simulink model "fmu_simulation"  (R2024a)
settings: Solver=ode1  StartTime=0.0  StopTime=200.0  FixedStep=0.01  RelTol=1e-3
settings Model: Creator=rkhan  LastModifiedBy=rkhan

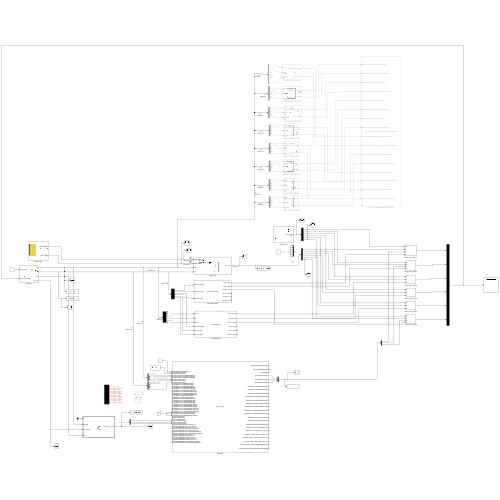
[thumbnail: Simulink's stored preview of the top-level diagram]
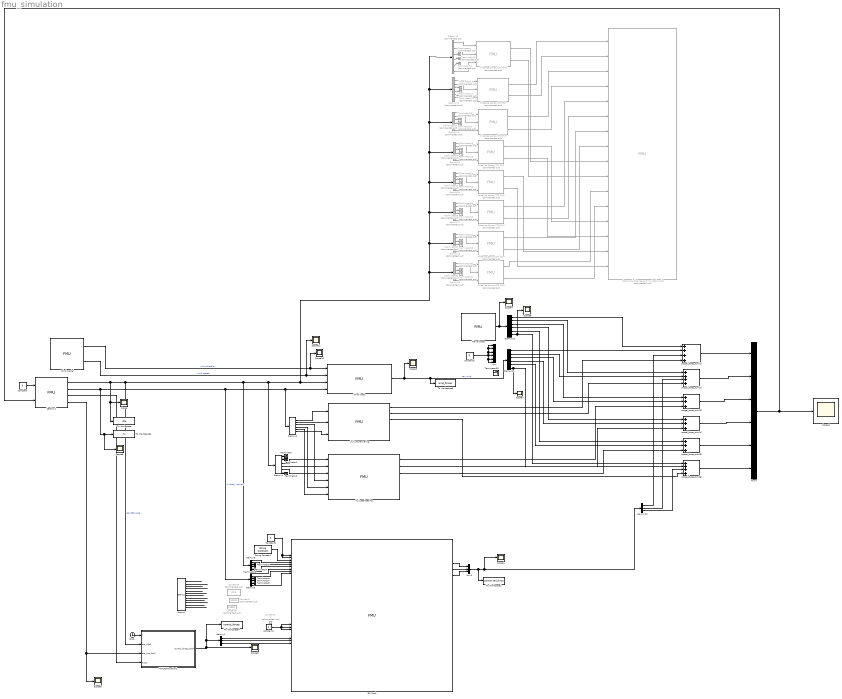
== system fmu_simulation ==
  Clock : Clock
  Constant : Constant  Value=0  OutDataTypeStr=boolean
  Constant1 : Constant  Value=0
  Constant2 : Constant  OutDataTypeStr=boolean
  Constant3 : Constant  Commented=on  Value=0
  Constant4 : Constant  OutDataTypeStr=double
  Constant6 : Constant  Commented=on  Value=3.0508
  Constant7 : Constant  Commented=on  Value=494.9
  Constant8 : Constant  Commented=on  Value=87.5
  DP Mock : FMU  FMUName=fmi_dp_mock.fmu  FMUMode=CoSimulation  FMUInitializeEnumObject=off  FMUCachedDialogLayout="{\"Geometry\":[471,-1082,1182,943],\"ParameterColumnsWidthConfig\":\"{\\\"columns\\\":[{\\\"name\\\":\\\"Parameter\\\",\\\"width\\\":422},{\\\"name\\\":\\\"Value\\\",\\\"width\\\":287},{\\\"name\\\":\\\"Unit\\\",\\\"width\\\":277},{\\\"name\\\":\\\"Description\\\",\\\"width\\\":339}]}\",\"InputColumnsWidthConfig\":[],\"OutputColumnsWidthConfig\":[]}"  Kp_0_=1485  Kp_1_=1800  Kp_2_=100000  Ki_0_=74  Ki_1_=90  Ki_2_=657  Kd_0_=19700  Kd_1_=23000  Kd_2_=173000  GeneralizedForcesSaturation_0_=10000  GeneralizedForcesSaturation_1_=10000  GeneralizedForcesSaturation_2_=35000  IntegralActionSaturation_0_=1000  IntegralActionSaturation_1_=1000  IntegralActionSaturation_2_=5000  MassMatrixDiagonal_0_=16500  MassMatrixDiagonal_1_=20000  MassMatrixDiagonal_2_=146000  DampingMatrixDiagonal_0_=100  DampingMatrixDiagonal_1_=1000  DampingMatrixDiagonal_2_=2200  MaxEffort_0_=5000  MaxEffort_1_=5000  MaxEffort_2_=5000  autopilot_heading_pid_Kp=70000  autopilot_heading_pid_Ki=0  autopilot_heading_pid_Kd=100000  autopilot_surge_speed_pid_Kp=3000  autopilot_surge_speed_pid_Ki=50  autopilot_surge_speed_pid_Kd=1000  mask(fmi_dp_mock [Co-Simulation, v2.0]){}
      mask Display:
      | disp('fmi_dp_mock');
      | port_label('output',1,'readyForAutonomyEnabled');
      | port_label('output',2,'autonomyModeEnabled');
      | port_label('output',3,'controlMode');
      | port_label('output',4,'generalizedForces[0]');
      | port_label('output',5,'generalizedForces[1]');
      | port_label('output',6,'generalizedForces[2]');
      | port_label('output',7,'refDPActive.northEastHeading[0]');
      | port_label('output',8,'refDPActive.northEastHeading[1]');
      | port_label('output',9,'refDPActive.northEastHeading[2]');
      | port_label('output',10,'refDPActive.northEastHeadingVel[0]');
      | port_label('output',11,'refDPActive.northEastHeadingVel[1]');
      | port_label('output',12,'refDPActive.northEastHeadingVel[2]');
      | port_label('output',13,'refDPActive.northEastHeadingAccel[0]');
      | port_label('output',14,'refDPActive.northEastHeadingAccel[1]');
      | port_label('output',15,'refDPActive.northEastHeadingAccel[2]');
      | port_label('output',16,'refDPActive.surgeIntegratorMode');
      | port_label('output',17,'refDPActive.swayIntegratorMode');
      | port_label('output',18,'refDPActive.headingIntegratorMode');
      | port_label('output',19,'autopilot_active_inputs.heading_ref');
      | port_label('output',20,'autopilot_active_inputs.yaw_rate_ref');
      | port_label('output',21,'autopilot_active_inputs.yaw_accel_ref');
      | port_label('output',22,'autopilot_active_inputs.surge_speed_ref');
      | port_label('output',23,'autopilot_active_inputs.surge_accel_ref');
      | port_label('output',24,'autopilot_active_inputs.surgeIntegratorMode');
      | port_label('output',25,'autopilot_active_inputs.headingIntegratorMode');
      | port_label('input',1,'enableReadyForAutonomy');
      | port_label('input',2,'enableAutonomyMode');
      | port_label('input',3,'desiredControlMode');
      | port_label('input',4,'measurements.northEastHeading[0]');
      | port_label('input',5,'measurements.northEastHeading[1]');
      | port_label('input',6,'measurements.northEastHeading[2]');
      | port_label('input',7,'measurements.nu[0]');
      | port_label('input',8,'measurements.nu[1]');
      | port_label('input',9,'measurements.nu[2]');
      | port_label('input',10,'refDpManual.northEastHeading[0]');
      | port_label('input',11,'refDpManual.northEastHeading[1]');
      | port_label('input',12,'refDpManual.northEastHeading[2]');
      | port_label('input',13,'refDpManual.northEastHeadingVel[0]');
      | port_label('input',14,'refDpManual.northEastHeadingVel[1]');
      | port_label('input',15,'refDpManual.northEastHeadingVel[2]');
      | port_label('input',16,'refDpManual.northEastHeadingAccel[0]');
      | port_label('input',17,'refDpManual.northEastHeadingAccel[1]');
      | port_label('input',18,'refDpManual.northEastHeadingAccel[2]');
      | port_label('input',19,'refDpManual.surgeIntegratorMode');
      | port_label('input',20,'refDpManual.swayIntegratorMode');
      | port_label('input',21,'refDpManual.headingIntegratorMode');
      | port_label('input',22,'refDpAutonomy.northEastHeading[0]');
      | port_label('input',23,'refDpAutonomy.northEastHeading[1]');
      | port_label('input',24,'refDpAutonomy.northEastHeading[2]');
      | port_label('input',25,'refDpAutonomy.northEastHeadingVel[0]');
      | port_label('input',26,'refDpAutonomy.northEastHeadingVel[1]');
      | port_label('input',27,'refDpAutonomy.northEastHeadingVel[2]');
      | port_label('input',28,'refDpAutonomy.northEastHeadingAccel[0]');
      | port_label('input',29,'refDpAutonomy.northEastHeadingAccel[1]');
      | port_label('input',30,'refDpAutonomy.northEastHeadingAccel[2]');
      | port_label('input',31,'refDpAutonomy.surgeIntegratorMode');
      | port_label('input',32,'refDpAutonomy.swayIntegratorMode');
      | port_label('input',33,'refDpAutonomy.headingIntegratorMode');
      | port_label('input',34,'refForcesManual[0]');
      | port_label('input',35,'refForcesManual[1]');
      | port_label('input',36,'refForcesManual[2]');
      | port_label('input',37,'refForcesAutonomy[0]');
      | port_label('input',38,'refForcesAutonomy[1]');
      | port_label('input',39,'refForcesAutonomy[2]');
      | port_label('input',40,'autopilotInputsAutonomy.heading_ref');
      | port_label('input',41,'autopilotInputsAutonomy.yaw_rate_ref');
      | port_label('input',42,'autopilotInputsAutonomy.yaw_accel_ref');
      | port_label('input',43,'autopilotInputsAutonomy.surge_speed_ref');
      | port_label('input',44,'autopilotInputsAutonomy.surge_accel_ref');
      | port_label('input',45,'autopilotInputsAutonomy.surgeIntegratorMode');
      | port_label('input',46,'autopilotInputsAutonomy.headingIntegratorMode');
      | port_label('input',47,'autopilotInputsManual.heading_ref');
      | port_label('input',48,'autopilotInputsManual.yaw_rate_ref');
      | port_label('input',49,'autopilotInputsManual.yaw_accel_ref');
      | port_label('input',50,'autopilotInputsManual.surge_speed_ref');
      | port_label('input',51,'autopilotInputsManual.surge_accel_ref');
      | port_label('input',52,'autopilotInputsManual.surgeIntegratorMode');
      | port_label('input',53,'autopilotInputsManual.headingIntegratorMode');
  Demux : Demux  Outputs=12
  Demux1 : Demux  Outputs=3
  Demux{12..19} (8 alike) : Demux  Commented=on  Outputs=6
  Demux{3..6,20..21} (6 alike) : Demux  Outputs=6
  Demux22 : Demux  Outputs=3
  Distance Sensor ZT1 FS-S : FMU  Commented=on  FMUName=UltrasonicDistanceSensor.fmu  FMUMode=CoSimulation  FMUCreateBusObject=off  FMUInitializeEnumObject=off  max_range=2  min_range=0.15  quay_1_depth=4.8  quay_1_p0=[81.7373060391681 498.883639455798]  quay_1_p1=[80.9216766435735 489.920674059846]  quay_2_depth=0.71  quay_2_p0=[93.6113480294073 496.95461073283]  quay_2_p1=[81.6607275014706 498.042116593623]  quay_3_depth=4.8  quay_3_p0=[619.016624410391 129.501263835181]  quay_3_p1=[618.965112725514 141.501153274102]  quay_4_depth=0.71  quay_4_p0=[606.991215224254 135.394697376503]  quay_4_p1=[618.991104663175 135.44620906138]  sensor_pose_psi=1.5708  sensor_pose_x=4.913  sensor_pose_y=2.4487  quay_1_en=on  quay_2_en=on  quay_3_en=on  quay_4_en=on  mask(UltrasonicDistanceSensor [Co-Simulation, v2.0]){}
      mask Display:
      | if (exist([Simulink.fileGenControl('get','CacheFolder') '\slprj\_fmu\777984f43c50f29a2c3e45720daf4c20\UltrasonicDistanceSensor\model.png'],'file'))
      |     image([Simulink.fileGenControl('get','CacheFolder') '\slprj\_fmu\777984f43c50f29a2c3e45720daf4c20\UltrasonicDistanceSensor\model.png']);
      | else
      |     disp('UltrasonicDistanceSensor');
      | end
      | port_label('output',1,'distance_measurement');
      | port_label('output',2,'signal_valid');
      | port_label('input',1,'north');
      | port_label('input',2,'east');
      | port_label('input',3,'heading');
  Distance Sensor ZT2 FS-F : FMU  Commented=on  FMUName=UltrasonicDistanceSensor_1.fmu  FMUMode=CoSimulation  FMUCreateBusObject=off  FMUInitializeEnumObject=off  max_range=2  min_range=0.15  quay_1_depth=4.8  quay_1_p0=[81.7373060391681 498.883639455798]  quay_1_p1=[80.9216766435735 489.920674059846]  quay_2_depth=0.71  quay_2_p0=[93.6113480294073 496.95461073283]  quay_2_p1=[81.6607275014706 498.042116593623]  quay_3_depth=4.8  quay_3_p0=[619.016624410391 129.501263835181]  quay_3_p1=[618.965112725514 141.501153274102]  quay_4_depth=0.71  quay_4_p0=[606.991215224254 135.394697376503]  quay_4_p1=[618.991104663175 135.44620906138]  sensor_pose_psi=0  sensor_pose_x=5.9479  sensor_pose_y=1.5  quay_1_en=on  quay_2_en=on  quay_3_en=on  quay_4_en=on  mask(UltrasonicDistanceSensor_1 [Co-Simulation, v2.0]){}
      mask Display:
      | if (exist([Simulink.fileGenControl('get','CacheFolder') '\slprj\_fmu\d35cb4a80b2d73ab213e5ce7f852a3cb\UltrasonicDistanceSensor_1\model.png'],'file'))
      |     image([Simulink.fileGenControl('get','CacheFolder') '\slprj\_fmu\d35cb4a80b2d73ab213e5ce7f852a3cb\UltrasonicDistanceSensor_1\model.png']);
      | else
      |     disp('UltrasonicDistanceSensor_1');
      | end
      | port_label('output',1,'distance_measurement');
      | port_label('output',2,'signal_valid');
      | port_label('input',1,'north');
      | port_label('input',2,'east');
      | port_label('input',3,'heading');
  Distance Sensor ZT3 FP-F : FMU  Commented=on  FMUName=UltrasonicDistanceSensor_2.fmu  FMUMode=CoSimulation  FMUCreateBusObject=off  FMUInitializeEnumObject=off  max_range=2  min_range=0.15  quay_1_depth=4.8  quay_1_p0=[81.7373060391681 498.883639455798]  quay_1_p1=[80.9216766435735 489.920674059846]  quay_2_depth=0.71  quay_2_p0=[93.6113480294073 496.95461073283]  quay_2_p1=[81.6607275014706 498.042116593623]  quay_3_depth=4.8  quay_3_p0=[619.016624410391 129.501263835181]  quay_3_p1=[618.965112725514 141.501153274102]  quay_4_depth=0.71  quay_4_p0=[606.991215224254 135.394697376503]  quay_4_p1=[618.991104663175 135.44620906138]  sensor_pose_psi=0  sensor_pose_x=5.9465  sensor_pose_y=-1.5  quay_1_en=on  quay_2_en=on  quay_3_en=on  quay_4_en=on  mask(UltrasonicDistanceSensor_2 [Co-Simulation, v2.0]){}
      mask Display:
      | if (exist([Simulink.fileGenControl('get','CacheFolder') '\slprj\_fmu\12532f91765f62f696db53de24741f0c\UltrasonicDistanceSensor_2\model.png'],'file'))
      |     image([Simulink.fileGenControl('get','CacheFolder') '\slprj\_fmu\12532f91765f62f696db53de24741f0c\UltrasonicDistanceSensor_2\model.png']);
      | else
      |     disp('UltrasonicDistanceSensor_2');
      | end
      | port_label('output',1,'distance_measurement');
      | port_label('output',2,'signal_valid');
      | port_label('input',1,'north');
      | port_label('input',2,'east');
      | port_label('input',3,'heading');
  Distance Sensor ZT4 FP-P : FMU  Commented=on  FMUName=UltrasonicDistanceSensor_3.fmu  FMUMode=CoSimulation  FMUCreateBusObject=off  FMUInitializeEnumObject=off  max_range=2  min_range=0.15  quay_1_depth=4.8  quay_1_p0=[81.7373060391681 498.883639455798]  quay_1_p1=[80.9216766435735 489.920674059846]  quay_2_depth=0.71  quay_2_p0=[93.6113480294073 496.95461073283]  quay_2_p1=[81.6607275014706 498.042116593623]  quay_3_depth=4.8  quay_3_p0=[619.016624410391 129.501263835181]  quay_3_p1=[618.965112725514 141.501153274102]  quay_4_depth=0.71  quay_4_p0=[606.991215224254 135.394697376503]  quay_4_p1=[618.991104663175 135.44620906138]  sensor_pose_psi=-1.5708  sensor_pose_x=4.913  sensor_pose_y=-2.4527  quay_1_en=on  quay_2_en=on  quay_3_en=on  quay_4_en=on  mask(UltrasonicDistanceSensor_3 [Co-Simulation, v2.0]){}
      mask Display:
      | if (exist([Simulink.fileGenControl('get','CacheFolder') '\slprj\_fmu\33e4b1bd19c1a4bbf282549265bfa70a\UltrasonicDistanceSensor_3\model.png'],'file'))
      |     image([Simulink.fileGenControl('get','CacheFolder') '\slprj\_fmu\33e4b1bd19c1a4bbf282549265bfa70a\UltrasonicDistanceSensor_3\model.png']);
      | else
      |     disp('UltrasonicDistanceSensor_3');
      | end
      | port_label('output',1,'distance_measurement');
      | port_label('output',2,'signal_valid');
      | port_label('input',1,'north');
      | port_label('input',2,'east');
      | port_label('input',3,'heading');
  Distance Sensor ZT5 AP-P : FMU  Commented=on  FMUName=UltrasonicDistanceSensor_4.fmu  FMUMode=CoSimulation  FMUCreateBusObject=off  FMUInitializeEnumObject=off  max_range=2  min_range=0.15  quay_1_depth=4.8  quay_1_p0=[81.7373060391681 498.883639455798]  quay_1_p1=[80.9216766435735 489.920674059846]  quay_2_depth=0.71  quay_2_p0=[93.6113480294073 496.95461073283]  quay_2_p1=[81.6607275014706 498.042116593623]  quay_3_depth=4.8  quay_3_p0=[619.016624410391 129.501263835181]  quay_3_p1=[618.965112725514 141.501153274102]  quay_4_depth=0.71  quay_4_p0=[606.991215224254 135.394697376503]  quay_4_p1=[618.991104663175 135.44620906138]  sensor_pose_psi=-1.5708  sensor_pose_x=-4.913  sensor_pose_y=-2.4514  quay_1_en=on  quay_2_en=on  quay_3_en=on  quay_4_en=on  mask(UltrasonicDistanceSensor_4 [Co-Simulation, v2.0]){}
      mask Display:
      | if (exist([Simulink.fileGenControl('get','CacheFolder') '\slprj\_fmu\2c6022cae16bfe16619e246ed39a73a9\UltrasonicDistanceSensor_4\model.png'],'file'))
      |     image([Simulink.fileGenControl('get','CacheFolder') '\slprj\_fmu\2c6022cae16bfe16619e246ed39a73a9\UltrasonicDistanceSensor_4\model.png']);
      | else
      |     disp('UltrasonicDistanceSensor_4');
      | end
      | port_label('output',1,'distance_measurement');
      | port_label('output',2,'signal_valid');
      | port_label('input',1,'north');
      | port_label('input',2,'east');
      | port_label('input',3,'heading');
  Distance Sensor ZT6 AP-A : FMU  Commented=on  FMUName=UltrasonicDistanceSensor_5.fmu  FMUMode=CoSimulation  FMUCreateBusObject=off  FMUInitializeEnumObject=off  max_range=2  min_range=0.15  quay_1_depth=4.8  quay_1_p0=[81.7373060391681 498.883639455798]  quay_1_p1=[80.9216766435735 489.920674059846]  quay_2_depth=0.71  quay_2_p0=[93.6113480294073 496.95461073283]  quay_2_p1=[81.6607275014706 498.042116593623]  quay_3_depth=4.8  quay_3_p0=[619.016624410391 129.501263835181]  quay_3_p1=[618.965112725514 141.501153274102]  quay_4_depth=0.71  quay_4_p0=[606.991215224254 135.394697376503]  quay_4_p1=[618.991104663175 135.44620906138]  sensor_pose_psi=3.1416  sensor_pose_x=-5.9427  sensor_pose_y=-1.5  quay_1_en=on  quay_2_en=on  quay_3_en=on  quay_4_en=on  mask(UltrasonicDistanceSensor_5 [Co-Simulation, v2.0]){}
      mask Display:
      | if (exist([Simulink.fileGenControl('get','CacheFolder') '\slprj\_fmu\5972c6e08933a554bbec62f557174caa\UltrasonicDistanceSensor_5\model.png'],'file'))
      |     image([Simulink.fileGenControl('get','CacheFolder') '\slprj\_fmu\5972c6e08933a554bbec62f557174caa\UltrasonicDistanceSensor_5\model.png']);
      | else
      |     disp('UltrasonicDistanceSensor_5');
      | end
      | port_label('output',1,'distance_measurement');
      | port_label('output',2,'signal_valid');
      | port_label('input',1,'north');
      | port_label('input',2,'east');
      | port_label('input',3,'heading');
  Distance Sensor ZT7 AS-A : FMU  Commented=on  FMUName=UltrasonicDistanceSensor_6.fmu  FMUMode=CoSimulation  FMUCreateBusObject=off  FMUInitializeEnumObject=off  max_range=2  min_range=0.15  quay_1_depth=4.8  quay_1_p0=[81.7373060391681 498.883639455798]  quay_1_p1=[80.9216766435735 489.920674059846]  quay_2_depth=0.71  quay_2_p0=[93.6113480294073 496.95461073283]  quay_2_p1=[81.6607275014706 498.042116593623]  quay_3_depth=4.8  quay_3_p0=[619.016624410391 129.501263835181]  quay_3_p1=[618.965112725514 141.501153274102]  quay_4_depth=0.71  quay_4_p0=[606.991215224254 135.394697376503]  quay_4_p1=[618.991104663175 135.44620906138]  sensor_pose_psi=3.1416  sensor_pose_x=-5.946  sensor_pose_y=1.5  quay_1_en=on  quay_2_en=on  quay_3_en=on  quay_4_en=on  mask(UltrasonicDistanceSensor_6 [Co-Simulation, v2.0]){}
      mask Display:
      | if (exist([Simulink.fileGenControl('get','CacheFolder') '\slprj\_fmu\76e2b9015701c0cf85d1e0a29a928fe7\UltrasonicDistanceSensor_6\model.png'],'file'))
      |     image([Simulink.fileGenControl('get','CacheFolder') '\slprj\_fmu\76e2b9015701c0cf85d1e0a29a928fe7\UltrasonicDistanceSensor_6\model.png']);
      | else
      |     disp('UltrasonicDistanceSensor_6');
      | end
      | port_label('output',1,'distance_measurement');
      | port_label('output',2,'signal_valid');
      | port_label('input',1,'north');
      | port_label('input',2,'east');
      | port_label('input',3,'heading');
  Distance Sensor ZT8 AS-S : FMU  Commented=on  FMUName=UltrasonicDistanceSensor_7.fmu  FMUMode=CoSimulation  FMUCreateBusObject=off  FMUInitializeEnumObject=off  max_range=2  min_range=0.15  quay_1_depth=4.8  quay_1_p0=[81.7373060391681 498.883639455798]  quay_1_p1=[80.9216766435735 489.920674059846]  quay_2_depth=0.71  quay_2_p0=[93.6113480294073 496.95461073283]  quay_2_p1=[81.6607275014706 498.042116593623]  quay_3_depth=4.8  quay_3_p0=[619.016624410391 129.501263835181]  quay_3_p1=[618.965112725514 141.501153274102]  quay_4_depth=0.71  quay_4_p0=[606.991215224254 135.394697376503]  quay_4_p1=[618.991104663175 135.44620906138]  sensor_pose_psi=1.5708  sensor_pose_x=-4.913  sensor_pose_y=2.4532  quay_1_en=on  quay_2_en=on  quay_3_en=on  quay_4_en=on  mask(UltrasonicDistanceSensor_7 [Co-Simulation, v2.0]){}
      mask Display:
      | if (exist([Simulink.fileGenControl('get','CacheFolder') '\slprj\_fmu\fcc687ec8d3596fcafe8ed7ad9aa01b3\UltrasonicDistanceSensor_7\model.png'],'file'))
      |     image([Simulink.fileGenControl('get','CacheFolder') '\slprj\_fmu\fcc687ec8d3596fcafe8ed7ad9aa01b3\UltrasonicDistanceSensor_7\model.png']);
      | else
      |     disp('UltrasonicDistanceSensor_7');
      | end
      | port_label('output',1,'distance_measurement');
      | port_label('output',2,'signal_valid');
      | port_label('input',1,'north');
      | port_label('input',2,'east');
      | port_label('input',3,'heading');
  MATLAB Function1 : MATLAB Function  TreatAsAtomicUnit=on
  Mux : Mux  Inputs=6
  Mux3 : Mux  Inputs=3
  Mux4 : Mux  Inputs=6
  Scope{,1..11} (12 alike) : Scope
  String Constant : StringConstant  String="\"JOYSTICK\""
  Terminator{,1..8,33} (10 alike) : Terminator
  Terminator{9..32} (24 alike) : Terminator  Commented=on
  To Workspace : ToWorkspace  VariableName=eta  SaveFormat=Timeseries  SampleTime=-1
  To Workspace1 : ToWorkspace  VariableName=generalized_forces  SaveFormat=Timeseries  SampleTime=-1
  To Workspace2 : ToWorkspace  VariableName=nu  SaveFormat=Timeseries  SampleTime=-1
  To Workspace3 : ToWorkspace  VariableName=wind_forces  SaveFormat=Structure With Time  SampleTime=-1
  To Workspace4 : ToWorkspace  VariableName=control_forces  SaveFormat=Timeseries  SampleTime=-1
  Wave forces : FMU  FMUName=wave_forces.fmu  FMUMode=CoSimulation  FMUCreateBusObject=off  FMUInitializeEnumObject=off  FMUCachedDialogLayout="{\"Geometry\":[99,-720,544,438],\"ParameterColumnsWidthConfig\":\"{\\\"columns\\\":[{\\\"name\\\":\\\"Parameter\\\",\\\"width\\\":219},{\\\"name\\\":\\\"Value\\\",\\\"width\\\":178},{\\\"name\\\":\\\"Unit\\\",\\\"width\\\":168},{\\\"name\\\":\\\"Description\\\",\\\"width\\\":231}]}\",\"InputColumnsWidthConfig\":[],\"OutputColumnsWidthConfig\":[]}"  wave_force_stddev=[0 0 0 0 0 0]  mask(wave_forces [Co-Simulation, v2.0]){}
      mask Display:
      | if (exist([Simulink.fileGenControl('get','CacheFolder') '\slprj\_fmu\fd9c0b8dd17c2899c609e22317adce66\wave_forces\model.png'],'file'))
      |     image([Simulink.fileGenControl('get','CacheFolder') '\slprj\_fmu\fd9c0b8dd17c2899c609e22317adce66\wave_forces\model.png']);
      | else
      |     disp('wave_forces');
      | end
      | port_label('output',1,'wave_forces');
  Wind loads : FMU  FMUName=wind_loads.fmu  FMUMode=CoSimulation  FMUCreateBusObject=off  FMUInitializeEnumObject=off  FMUCachedDialogLayout="{\"Geometry\":[-706,310,544,438],\"ParameterColumnsWidthConfig\":\"{\\\"columns\\\":[{\\\"name\\\":\\\"Parameter\\\",\\\"width\\\":213},{\\\"name\\\":\\\"Value\\\",\\\"width\\\":172},{\\\"name\\\":\\\"Unit\\\",\\\"width\\\":162},{\\\"name\\\":\\\"Description\\\",\\\"width\\\":223}]}\",\"InputColumnsWidthConfig\":[],\"OutputColumnsWidthConfig\":[]}"  A_Fw=19  A_Lw=45.6  CD_lAF=0.475  CD_t=0.9  H_Lw=1  L_oa=12  delta=0.8  kappa=1.1  rho_air=1.225  s_L=0  mask(wind_loads [Co-Simulation, v2.0]){}
      mask Display:
      | if (exist([Simulink.fileGenControl('get','CacheFolder') '\slprj\_fmu\d2b23ac574a1a1755c9ff6305b322350\wind_loads\model.png'],'file'))
      |     image([Simulink.fileGenControl('get','CacheFolder') '\slprj\_fmu\d2b23ac574a1a1755c9ff6305b322350\wind_loads\model.png']);
      | else
      |     disp('wind_loads');
      | end
      | port_label('output',1,'tau_wind');
      | port_label('input',1,'wind_direction');
      | port_label('input',2,'wind_speed');
      | port_label('input',3,'eta');
      | port_label('input',4,'nu');
  Wind model : FMU  FMUName=wind_model.fmu  FMUMode=CoSimulation  FMUCreateBusObject=off  FMUInitializeEnumObject=off  FMUCachedDialogLayout="{\"Geometry\":[-374,-868,1009,511],\"ParameterColumnsWidthConfig\":\"{\\\"columns\\\":[{\\\"name\\\":\\\"Parameter\\\",\\\"width\\\":393},{\\\"name\\\":\\\"Value\\\",\\\"width\\\":352},{\\\"name\\\":\\\"Unit\\\",\\\"width\\\":342},{\\\"name\\\":\\\"Description\\\",\\\"width\\\":406}]}\",\"InputColumnsWidthConfig\":[],\"OutputColumnsWidthConfig\":[]}"  mean_wind_direction=4.62163884  mean_wind_speed=11  wind_direction_noise_power=0  wind_direction_time_constant=10  wind_speed_noise_power=0  wind_speed_time_constant=10  mask(wind_model [Co-Simulation, v2.0]){}
      mask Display:
      | if (exist([Simulink.fileGenControl('get','CacheFolder') '\slprj\_fmu\c187fdecdb54de7a5e69be10c905a05b\wind_model\model.png'],'file'))
      |     image([Simulink.fileGenControl('get','CacheFolder') '\slprj\_fmu\c187fdecdb54de7a5e69be10c905a05b\wind_model\model.png']);
      | else
      |     disp('wind_model');
      | end
      | port_label('output',1,'wind_direction');
      | port_label('output',2,'wind_speed');
  Zeabuz 1 : FMU  FMUName=rigid_body.fmu  FMUMode=CoSimulation  FMUCreateBusObject=off  FMUInitializeEnumObject=off  FMUCachedDialogLayout="{\"Geometry\":[-527,-948,1072,799],\"ParameterColumnsWidthConfig\":\"{\\\"columns\\\":[{\\\"name\\\":\\\"Parameter\\\",\\\"width\\\":529},{\\\"name\\\":\\\"Value\\\",\\\"width\\\":169},{\\\"name\\\":\\\"Unit\\\",\\\"width\\\":478},{\\\"name\\\":\\\"Description\\\",\\\"width\\\":540}]}\",\"InputColumnsWidthConfig\":[],\"OutputColumnsWidthConfig\":[]}"  B_vessel=5.25  I=[49357 145050 145050]  I_added=[24679 0 4497.2821]  L_vessel=12.25  d_quay=160000  initial_position=[130 470 0 0 0 2.4]  initial_velocity=[1 0 0 0 0 0]  k_quay=100000  m=16116.7  m_added=[805.835 16116.7 8058]  mu_quay=1  quay_1_depth=4.8  quay_1_p0=[81.7373060391681 498.883639455798]  quay_1_p1=[80.9216766435735 489.920674059846]  quay_2_depth=0.71  quay_2_p0=[93.6113480294073 496.95461073283]  quay_2_p1=[81.6607275014706 498.042116593623]  quay_3_depth=4.8  quay_3_p0=[619.016624410391 129.501263835181]  quay_3_p1=[618.965112725514 141.501153274102]  quay_4_depth=0.71  quay_4_p0=[606.991215224254 135.394697376503]  quay_4_p1=[618.991104663175 135.44620906138]  quay_1_en=on  quay_2_en=on  quay_3_en=off  quay_4_en=off  mask(rigid_body [Co-Simulation, v2.0]){}
      mask Display:
      | if (exist([Simulink.fileGenControl('get','CacheFolder') '\slprj\_fmu\a830fc9151b88ce01983342fe088bcac\rigid_body\model.png'],'file'))
      |     image([Simulink.fileGenControl('get','CacheFolder') '\slprj\_fmu\a830fc9151b88ce01983342fe088bcac\rigid_body\model.png']);
      | else
      |     disp('rigid_body');
      | end
      | port_label('output',1,'eta');
      | port_label('output',2,'nu');
      | port_label('output',3,'acc');
      | port_label('output',4,'eta_dot');
      | port_label('input',1,'lock_motion');
      | port_label('input',2,'external_force');
  hull_maneuvering : FMU  FMUName=hull_maneuvering.fmu  FMUMode=CoSimulation  FMUInitializeEnumObject=off  density=1025.9  kinematic_viscosity=0.00000119  length=12  depth=0.91  wetted_surface=46.41  shape_factor=0.052  CR_m=4.105  CR_p=5.8  CD_lateral=0  Xvv=-0.04  Xvr=0.002  Xrr=0.011  Xvvvv=0.771  Yv=-0.315  Yr=0.083  Yvvv=-1.607  Yvvr=0.379  Yvrr=-0.391  Yrrr=0.008  Nv=-0.137  Nr=-0.049  Nvvv=-0.03  Nvvr=-0.294  Nvrr=0.055  Nrrr=-0.013  CX_low=0.05  CY_low=0.5  CN_low=0.11051  Nr_low=-5000  speed_limit_low=0.5  speed_transfer_range=0.2572  low_speed_model=on  high_speed_model=on  mask(hull_maneuvering [Co-Simulation, v2.0]){}
      mask Display:
      | disp('hull_maneuvering');
      | port_label('output',1,'force_surge');
      | port_label('output',2,'force_sway');
      | port_label('output',3,'moment_yaw');
      | port_label('output',4,'force_heave');
      | port_label('output',5,'moment_roll');
      | port_label('output',6,'moment_pitch');
      | port_label('input',1,'velocity_surge');
      | port_label('input',2,'velocity_sway');
      | port_label('input',3,'velocity_yaw');
  hull_seakeeping : FMU  FMUName=hull_seakeeping.fmu  FMUMode=CoSimulation  FMUInitializeEnumObject=off  density=1025.9  gravity=9.81  heave_damping=46418.3301  roll_damping=60895.7369  pitch_damping=303539.5095  GM_roll=3.52  GM_pitch=11.16  mass=16116.7  waterplane_area=24.6  mask(hull_seakeeping [Co-Simulation, v2.0]){}
      mask Display:
      | disp('hull_seakeeping');
      | port_label('output',1,'force_heave');
      | port_label('output',2,'moment_roll');
      | port_label('output',3,'moment_pitch');
      | port_label('output',4,'force_surge');
      | port_label('output',5,'force_sway');
      | port_label('output',6,'moment_yaw');
      | port_label('input',1,'heave');
      | port_label('input',2,'roll');
      | port_label('input',3,'pitch');
      | port_label('input',4,'velocity_heave');
      | port_label('input',5,'velocity_roll');
      | port_label('input',6,'velocity_pitch');
  ultrasound_distance_communication_zb1 : FMU  Commented=on  FMUName=fmi_ultrasonic_distance_sensor_communication_zb1.fmu  FMUMode=CoSimulation  FMUInitializeEnumObject=off  remote_ip=127.0.0.1  local_ip=0.0.0.0  remote_port=2001  local_port=1996  dump_messages=off  mask(fmi_ultrasonic_distance_sensor_communication_zb1 [Co-Simulation, v2.0]){}
      mask Display:
      | disp('fmi_ultrasonic_distance_sensor_communication_zb1');
      | port_label('input',1,'ultrasonic_dist_fore_stbd_measurement');
      | port_label('input',2,'ultrasonic_dist_fore_stbd_measurement_valid');
      | port_label('input',3,'ultrasonic_dist_fore_port_measurement');
      | port_label('input',4,'ultrasonic_dist_fore_port_measurement_valid');
      | port_label('input',5,'ultrasonic_dist_aft_port_measurement');
      | port_label('input',6,'ultrasonic_dist_aft_port_measurement_valid');
      | port_label('input',7,'ultrasonic_dist_aft_stbd_measurement');
      | port_label('input',8,'ultrasonic_dist_aft_stbd_measurement_valid');
      | port_label('input',9,'ultrasonic_dist_alongside_fore_stbd_measurement');
      | port_label('input',10,'ultrasonic_dist_alongside_fore_stbd_measurement_valid');
      | port_label('input',11,'ultrasonic_dist_alongside_aft_stbd_measurement');
      | port_label('input',12,'ultrasonic_dist_alongside_aft_stbd_measurement_valid');
      | port_label('input',13,'ultrasonic_dist_alongside_fore_port_measurement');
      | port_label('input',14,'ultrasonic_dist_alongside_fore_port_measurement_valid');
      | port_label('input',15,'ultrasonic_dist_alongside_aft_port_measurement');
      | port_label('input',16,'ultrasonic_dist_alongside_aft_port_measurement_valid');
  vessel_force_sum[1] : Sum  Inputs=++++
  vessel_force_sum[2] : Sum  Inputs=++++
  vessel_force_sum[3] : Sum  Inputs=+++
  vessel_force_sum[4] : Sum  Inputs=+++
  vessel_force_sum[5] : Sum  Inputs=+++
  vessel_force_sum[6] : Sum  Inputs=++++
  wires:
  Wind model/1 -> Scope10/1, Wind loads/1  "wind direction"
  Wind model/2 -> Scope11/1, Wind loads/2  "wind speed"
  Zeabuz 1/1 -> To Workspace/1, Scope/1, Demux5/1, Wind loads/3, Demux19/1, Demux16/1, Demux15/1, Demux13/1, Demux12/1, Demux14/1, Demux17/1, Demux18/1, Demux4/1, MATLAB Function1/2(eta_6dof)  "eta NED pose"
  Zeabuz 1/2 -> Scope6/1, To Workspace2/1, Wind loads/4, Demux3/1, Demux6/1  "nu body velocity"
  Demux/1 -> ?
  Demux/2 -> ?
  Demux/3 -> ?
  Demux/4 -> ?
  Demux/5 -> ?
  Demux/6 -> ?
  Demux/7 -> ?
  Demux/8 -> ?
  Demux/9 -> ?
  Demux/10 -> ?
  Demux/11 -> ?
  Demux/12 -> ?
  Demux5/1 -> DP Mock/4
  Demux5/2 -> DP Mock/5
  Demux5/6 -> DP Mock/6
  Demux6/1 -> DP Mock/7
  Demux6/2 -> DP Mock/8
  Demux6/6 -> DP Mock/9
  Demux5/3 -> Terminator3/1
  Demux5/4 -> Terminator4/1
  Demux5/5 -> Terminator5/1
  Demux6/3 -> Terminator6/1
  Demux6/4 -> Terminator7/1
  Demux6/5 -> Terminator8/1
  Demux12/1 -> Distance Sensor ZT1 FS-S/1
  Demux12/2 -> Distance Sensor ZT1 FS-S/2
  Demux12/6 -> Distance Sensor ZT1 FS-S/3
  Demux12/3 -> Terminator9/1
  Demux12/4 -> Terminator10/1
  Demux12/5 -> Terminator11/1
  Demux13/5 -> Terminator13/1
  Demux13/4 -> Terminator12/1
  Demux13/3 -> Terminator14/1
  Demux13/6 -> Distance Sensor ZT2 FS-F/3
  Demux13/2 -> Distance Sensor ZT2 FS-F/2
  Demux13/1 -> Distance Sensor ZT2 FS-F/1
  Demux14/1 -> Distance Sensor ZT3 FP-F/1
  Demux14/2 -> Distance Sensor ZT3 FP-F/2
  Demux14/6 -> Distance Sensor ZT3 FP-F/3
  Demux14/3 -> Terminator15/1
  Demux14/4 -> Terminator16/1
  Demux14/5 -> Terminator17/1
  Demux15/6 -> Distance Sensor ZT4 FP-P/3
  Demux15/4 -> Terminator19/1
  Demux15/1 -> Distance Sensor ZT4 FP-P/1
  Demux15/2 -> Distance Sensor ZT4 FP-P/2
  Demux15/5 -> Terminator20/1
  Demux15/3 -> Terminator18/1
  Demux16/6 -> Distance Sensor ZT5 AP-P/3
  Demux16/4 -> Terminator22/1
  Demux16/1 -> Distance Sensor ZT5 AP-P/1
  Demux16/2 -> Distance Sensor ZT5 AP-P/2
  Demux16/5 -> Terminator23/1
  Demux16/3 -> Terminator21/1
  Demux17/6 -> Distance Sensor ZT6 AP-A/3
  Demux17/4 -> Terminator25/1
  Demux17/1 -> Distance Sensor ZT6 AP-A/1
  Demux17/2 -> Distance Sensor ZT6 AP-A/2
  Demux17/5 -> Terminator26/1
  Demux17/3 -> Terminator24/1
  Demux18/6 -> Distance Sensor ZT7 AS-A/3
  Demux18/4 -> Terminator28/1
  Demux18/1 -> Distance Sensor ZT7 AS-A/1
  Demux18/2 -> Distance Sensor ZT7 AS-A/2
  Demux18/5 -> Terminator29/1
  Demux18/3 -> Terminator27/1
  Demux19/6 -> Distance Sensor ZT8 AS-S/3
  Demux19/4 -> Terminator31/1
  Demux19/1 -> Distance Sensor ZT8 AS-S/1
  Demux19/2 -> Distance Sensor ZT8 AS-S/2
  Demux19/5 -> Terminator32/1
  Demux19/3 -> Terminator30/1
  Distance Sensor ZT1 FS-S/1 -> ultrasound_distance_communication_zb1/9
  Distance Sensor ZT1 FS-S/2 -> ultrasound_distance_communication_zb1/10
  Distance Sensor ZT2 FS-F/1 -> ultrasound_distance_communication_zb1/1
  Distance Sensor ZT2 FS-F/2 -> ultrasound_distance_communication_zb1/2
  Distance Sensor ZT3 FP-F/1 -> ultrasound_distance_communication_zb1/3
  Distance Sensor ZT3 FP-F/2 -> ultrasound_distance_communication_zb1/4
  Distance Sensor ZT4 FP-P/1 -> ultrasound_distance_communication_zb1/13
  Distance Sensor ZT4 FP-P/2 -> ultrasound_distance_communication_zb1/14
  Distance Sensor ZT5 AP-P/1 -> ultrasound_distance_communication_zb1/15
  Distance Sensor ZT5 AP-P/2 -> ultrasound_distance_communication_zb1/16
  Distance Sensor ZT6 AP-A/1 -> ultrasound_distance_communication_zb1/5
  Distance Sensor ZT6 AP-A/2 -> ultrasound_distance_communication_zb1/6
  Distance Sensor ZT7 AS-A/1 -> ultrasound_distance_communication_zb1/7
  Distance Sensor ZT7 AS-A/2 -> ultrasound_distance_communication_zb1/8
  Distance Sensor ZT8 AS-S/1 -> ultrasound_distance_communication_zb1/11
  Distance Sensor ZT8 AS-S/2 -> ultrasound_distance_communication_zb1/12
  Demux20/1 -> vessel_force_sum[1]/1
  Demux21/1 -> vessel_force_sum[1]/2
  hull_maneuvering/1 -> vessel_force_sum[1]/4
  DP Mock/4 -> Mux3/1
  DP Mock/5 -> Mux3/2
  DP Mock/6 -> Mux3/3
  Mux3/1 -> To Workspace1/1, Scope1/1, Demux22/1
  Demux22/1 -> vessel_force_sum[1]/3
  Demux20/2 -> vessel_force_sum[2]/1
  Demux21/2 -> vessel_force_sum[2]/2
  Demux22/2 -> vessel_force_sum[2]/3
  hull_maneuvering/2 -> vessel_force_sum[2]/4
  Demux20/3 -> vessel_force_sum[3]/1
  Demux21/3 -> vessel_force_sum[3]/2
  hull_seakeeping/1 -> vessel_force_sum[3]/3
  Demux20/4 -> vessel_force_sum[4]/1
  Demux21/4 -> vessel_force_sum[4]/2
  hull_seakeeping/2 -> vessel_force_sum[4]/3
  Demux20/5 -> vessel_force_sum[5]/1
  Demux21/5 -> vessel_force_sum[5]/2
  hull_seakeeping/3 -> vessel_force_sum[5]/3
  Demux20/6 -> Scope8/1, vessel_force_sum[6]/1
  Demux21/6 -> vessel_force_sum[6]/2, Scope7/1
  Demux22/3 -> vessel_force_sum[6]/3
  hull_maneuvering/3 -> vessel_force_sum[6]/4
  vessel_force_sum[1]/1 -> Mux4/1
  vessel_force_sum[2]/1 -> Mux4/2
  vessel_force_sum[3]/1 -> Mux4/3
  vessel_force_sum[4]/1 -> Mux4/4
  vessel_force_sum[5]/1 -> Mux4/5
  vessel_force_sum[6]/1 -> Mux4/6
  Mux4/1 -> Zeabuz 1/2, Scope2/1
  Constant/1 -> Zeabuz 1/1
  Constant2/1 -> DP Mock/2, DP Mock/1
  String Constant/1 -> DP Mock/3
  Demux3/3 -> hull_seakeeping/4
  Demux3/4 -> hull_seakeeping/5
  Demux3/5 -> hull_seakeeping/6
  Demux4/3 -> hull_seakeeping/1
  Demux4/4 -> hull_seakeeping/2
  Demux4/5 -> hull_seakeeping/3
  Demux3/1 -> hull_maneuvering/1
  Demux3/2 -> hull_maneuvering/2
  Demux3/6 -> hull_maneuvering/3
  Demux4/1 -> Terminator/1
  Demux4/2 -> Terminator1/1
  Demux4/6 -> Terminator2/1
  Constant4/1 -> DP Mock/31, DP Mock/32, DP Mock/33
  Demux1/1 -> DP Mock/37
  Demux1/2 -> DP Mock/38
  Demux1/3 -> DP Mock/39
  Zeabuz 1/4 -> Scope5/1, MATLAB Function1/3(eta_dot_6dof)
  MATLAB Function1/1(control_forces_3dof) -> To Workspace4/1, Demux1/1, Scope3/1
  Clock/1 -> MATLAB Function1/1(t)
  Wave forces/1 -> Demux20/1, Scope4/1
  Wind loads/1 -> Demux21/1, To Workspace3/1, Scope9/1  "tau wind"
  Zeabuz 1/3 -> MATLAB Function1/4(accel)
  Constant1/1 -> Mux/6, Mux/5, Mux/1, Mux/2, Mux/3, Mux/4

== matlab function fmu_simulation/MATLAB Function1 ==
  data: t input; eta_6dof input; control_forces_3dof output; eta_dot_6dof input; accel input
function control_forces_3dof  = extended_dp_docking(t, eta_6dof, eta_dot_6dof, accel)
    % This function calls the 'run' method in the Python docking algorithm package.
    coder.extrinsic('docking_wrapper');
    % coder.extrinsic('set_fmu_parameters_for_run');


    % SET THE FOLLOWING PARAMETERS BEFORE EACH RUN !!!
    % batch = "no_disturbances"; % options: "no_disturbances, small_disturbances, moderate_disturbances, large_disturbances
    % run = 1;
    % quay_type = "l_quay";  % options: l_quay, h_quay
    % controller_type = "pid"; % options: pid, mpc 
    % run_description = '';
    % if ~isempty(run_description)
    %     output_filepath = fullfile('../../masteroppgave-rapport/results', controller_type, batch, strcat('run', num2str(run)), run_description, 'fmu_params.csv');
    % else
    %     output_filepath = fullfile('../../masteroppgave-rapport/results', controller_type, batch, strcat('run', num2str(run)), 'fmu_params.csv');
    % end
    % 
    % 
    % 
    % if quay_type == "l_quay"
    %     enable_l = 1;
    % else
    %     enable_l = 0;
    % end
    % 
    % % FMU parameters
    % fmuParams = struct(...
    %     'WindModel', struct('mean_wind_direction', 0, 'wind_direction_noise_power', 0, 'wind_direction_time_constant', 10,...
    %                         'mean_wind_speed', 0, 'wind_speed_noise_power', 0, 'wind_speed_time_constant', 10),...
    %     'WaveForces', struct('wave_force_stddev', [0, 0, 0, 0, 0, 0]), ...
    %     'Zeabuz', struct('initial_position', [100, 484, 0, 0, 0, 2.42], 'initial_velocity', [0.3, 0, 0, 0, 0, 0], 'quay_1_en', 1, 'quay_2_en', enable_l),...
    %     'DistanceSensorZT1FSS', struct('quay_1_en', 1, 'quay_2_en', enable_l),...
    %     'DistanceSensorZT2FSF', struct('quay_1_en', 1, 'quay_2_en', enable_l),...
    %     'DistanceSensorZT3FPF', struct('quay_1_en', 1, 'quay_2_en', enable_l),...
    %     'DistanceSensorZT4FPP', struct('quay_1_en', 1, 'quay_2_en', enable_l),...
    %     'DistanceSensorZT5APP', struct('quay_1_en', 1, 'quay_2_en', enable_l),...
    %     'DistanceSensorZT6APA', struct('quay_1_en', 1, 'quay_2_en', enable_l),...
    %     'DistanceSensorZT7ASA', struct('quay_1_en', 1, 'quay_2_en', enable_l),...
    %     'DistanceSensorZT8ASS', struct('quay_1_en', 1, 'quay_2_en', enable_l)...
    % );



    % Define the 10 Hz execution interval
    exec_interval = 0.1;  % 10 Hz = 0.1 second interval

    % Declare persistent variables to store previous output and prev execution time
    persistent prev_control_forces prev_exec_time; % fmu_initialized;

    % if isempty(fmu_initialized)
    %     fmu_initialized = false;
    % end

    if isempty(prev_exec_time)
        prev_exec_time = t;  % Initialize prev execution time
    end

    % Initialize persistent variables on the first call
    if isempty(prev_control_forces)
        eta_3dof = [eta_6dof(1), eta_6dof(2), eta_6dof(6)];
        eta_dot_3dof = [eta_dot_6dof(1), eta_dot_6dof(2), eta_dot_6dof(6)];
    
        control_forces_3dof = zeros(size(eta_3dof));  % initializing
        prev_control_forces = zeros(size(eta_3dof));  % initializing

        % [control_forces_3dof, eta_d_3dof] = docking_wrapper(t, eta_3dof, eta_dot_3dof, accel, batch, run, controller_type, quay_type, run_description);
        control_forces_3dof = docking_wrapper(t, eta_3dof, eta_dot_3dof, accel);

        prev_control_forces = control_forces_3dof;

        % if ~fmu_initialized
        %     set_fmu_parameters_for_run(fmuParams, output_filepath);  % Call the external function
        %     fmu_initialized = true;  % Ensure it runs only once
        % end

    end


    % Check if it's time to execute the function (every 0.1s)
    if t >= prev_exec_time + exec_interval
        % Run the docking_wrapper function every 0.1 seconds
        eta_3dof = [eta_6dof(1), eta_6dof(2), eta_6dof(6)];
        eta_dot_3dof = [eta_dot_6dof(1), eta_dot_6dof(2), eta_dot_6dof(6)];

        %control_forces_3dof = zeros(size(eta_3dof));  % initializing
        % [control_forces_3dof, eta_d_3dof] = docking_wrapper(t, eta_3dof, eta_dot_3dof, accel, batch, run, controller_type, quay_type, run_description);
        control_forces_3dof = docking_wrapper(t, eta_3dof, eta_dot_3dof, accel);
        
        % Update the prev output and the prev execution time
        prev_control_forces = control_forces_3dof;
        prev_exec_time = t;
    else
        % If it's not time to execute, output the previous control forces
        control_forces_3dof = prev_control_forces;
    end
end
